simulink model "model_simulink"  (R2023b)
settings: Solver=VariableStepAuto  StartTime=0.0  StopTime=60  RelTol=1e-3
values from neighbouring files (symbols this model uses):
  x0 = [alpha(i)+theta1_init; theta2_init; 0; 0]    [tema1_ms.m]
settings Model: Creator=Ioana  LastModifiedBy=Ioana

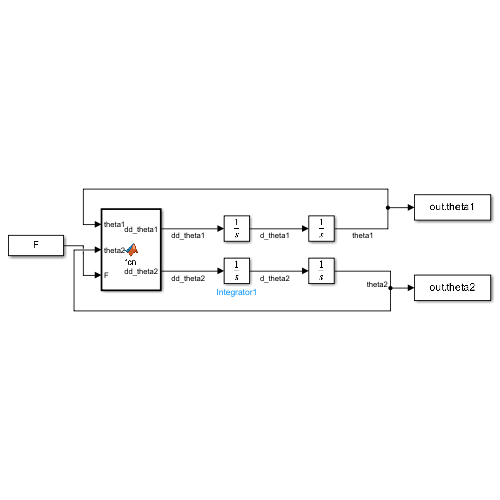
[thumbnail: Simulink's stored preview of the top-level diagram]
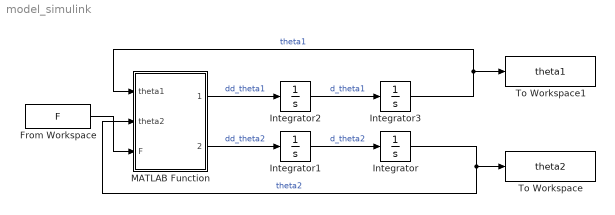
== system model_simulink ==
  From Workspace : FromWorkspace  VariableName=F
  Integrator : Integrator  InitialCondition=x0(2)
  Integrator1 : Integrator
  Integrator2 : Integrator
  Integrator3 : Integrator  InitialCondition=x0(1)
  MATLAB Function : MATLAB Function  TreatAsAtomicUnit=on
  To Workspace : ToWorkspace  VariableName=theta2  SaveFormat=Timeseries  SampleTime=-1
  To Workspace1 : ToWorkspace  VariableName=theta1  SaveFormat=Timeseries  SampleTime=-1
  wires:
  Integrator1/1 -> Integrator/1  "d_theta2"
  MATLAB Function/2(dd_theta2) -> Integrator1/1  "dd_theta2"
  MATLAB Function/1(dd_theta1) -> Integrator2/1  "dd_theta1"
  Integrator2/1 -> Integrator3/1  "d_theta1"
  Integrator3/1 -> To Workspace1/1, MATLAB Function/1(theta1)  "theta1"
  Integrator/1 -> MATLAB Function/2(theta2), To Workspace/1  "theta2"
  From Workspace/1 -> MATLAB Function/3(F)

== matlab function model_simulink/MATLAB Function ==
  data: theta1 input; theta2 input; F input; dd_theta1 output; dd_theta2 output
function [dd_theta1,dd_theta2]= fcn(theta1, theta2,F)


M=1;
L=1;
g=9.81;
k=100;

dd_theta1=(F-M*g*L*sin(theta1)-1/4*k*(L^2)*(sin(theta1)-sin(theta2))*cos(theta1))/(M*L^2);

dd_theta2=(-M*g*L*sin(theta2)+1/4*k*(L^2)*(sin(theta1)-sin(theta2))*cos(theta2))/(M*L^2);
